simulink model "ParameterEstimation_SimplePendulum"  (R2015b)
settings: Solver=FixedStepAuto  SolverMode=SingleTasking  StartTime=0.0  StopTime=40  FixedStep=T  RelTol=1e-3
values from neighbouring files (symbols this model uses):
  datainit = 1.58997108664    [realVSmodel_fwAnd5vstepsx3AndChirp_outerSW.mat]
  J = 4.37484748956    [realVSmodel_fwAnd5vstepsx3AndChirp_outerSW.mat]
  Kt = 18.3    [realVSmodel_fwAnd5vstepsx3AndChirp_outerSW.mat]
undefined symbols (not defined in the file or in its folder): Fv, g, lc, m
libraries: simulink x1
settings Model: Creator=mounir  LastModifiedBy=mounir
settings DataIOCC: SaveFormat=Array
settings OptimizationCC: BlockReduction=off  BooleanDataType=off  ExpressionDepthLimit=2147483647
settings DebuggingCC: SaveWithParameterizedLinksMsg=none  UnderspecifiedInitializationDetection=Classic  MergeDetectMultiDrivingBlocksExec=none  SignalResolutionControl=TryResolveAllWithWarning  MultiTaskDSMMsg=warning  MultiTaskCondExecSysMsg=none  StateNameClashWarn=warning
settings HardwareCC: ProdBitPerPointer=32  ProdLargestAtomicFloat=None  ProdIntDivRoundTo=Undefined  ProdEndianess=Unspecified  ProdWordSize=32  ProdHWDeviceType=32-bit Generic  TargetUnknown=on
settings GRTTargetCC: GeneratePreprocessorConditionals=Disable all
settings ConfigComp: CovModelRefEnable=Off

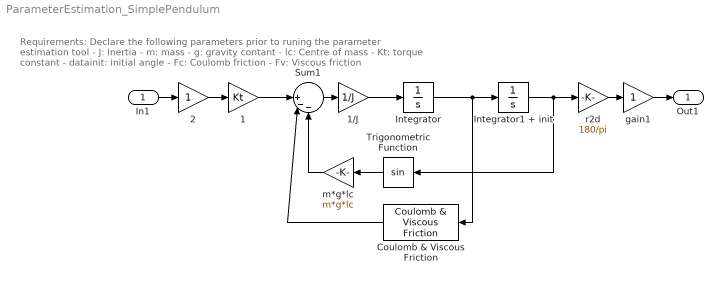
== system ParameterEstimation_SimplePendulum ==
  note: Requirements:
      | Declare the following parameters prior to runing the parameter estimation tool
      |  - J: Inertia
      |  - m: mass
      |  - g: gravity contant
      |  - lc: Centre of mass
      |  - Kt: torque constant
      |  - datainit: initial angle
      |  - Fc: Coulomb friction
      |  - Fv: Viscous friction
  In1 : Inport
  1 : Gain  Gain=Kt
  1/J : Gain  Gain=1/J
  2 : Gain
  Coulomb & Viscous Friction : simulink/Discontinuities/Coulomb & Viscous Friction  offset=Fc  gain=Fv
  Integrator : Integrator
  Integrator1 + init : Integrator  InitialCondition=datainit
  Sum1 : Sum  Inputs=||+--
  Trigonometric Function : Trigonometry
  gain1 : Gain
  m*g*lc : Gain  Gain=m*g*lc
  r2d : Gain  Gain=180/pi
  Out1 : Outport
  wires:
  In1/1 -> 2/1
  Sum1/1 -> 1/J/1
  1/1 -> Sum1/1
  Integrator/1 -> Coulomb & Viscous Friction/1, Integrator1 + init/1
  Trigonometric Function/1 -> m*g*lc/1
  m*g*lc/1 -> Sum1/3
  1/J/1 -> Integrator/1
  Coulomb & Viscous Friction/1 -> Sum1/2
  Integrator1 + init/1 -> r2d/1, Trigonometric Function/1
  r2d/1 -> gain1/1
  2/1 -> 1/1
  gain1/1 -> Out1/1
